simulink model "variacion_tau"  (R2026a)
settings: Solver=VariableStepAuto
values from neighbouring files (symbols this model uses):
  K = cambio_y / delta_u    [Taller_1_Identificacion_grafica_de_sistemas_FOTD.m]
  t_escalon = t(idx_escalon + 1)    [Taller_1_Identificacion_grafica_de_sistemas_FOTD.m]
  tau_analitico = 1.5 * (t_63_relativo - t_28_relativo)    [Taller_1_Identificacion_grafica_de_sistemas_FOTD.m]
  theta_analitico = t_63_relativo - tau_analitico    [Taller_1_Identificacion_grafica_de_sistemas_FOTD.m]
settings Model: Creator=Daniel  LastModifiedBy=Daniel

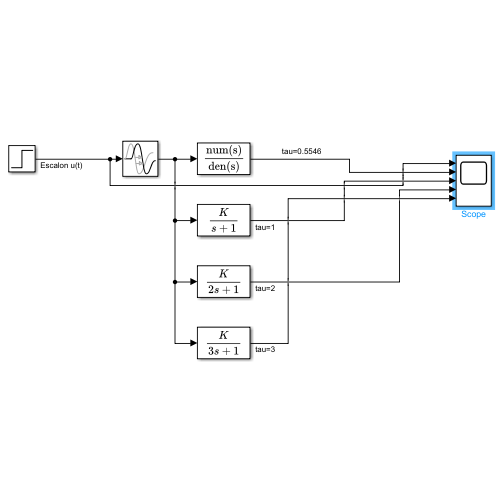
[thumbnail: Simulink's stored preview of the top-level diagram]
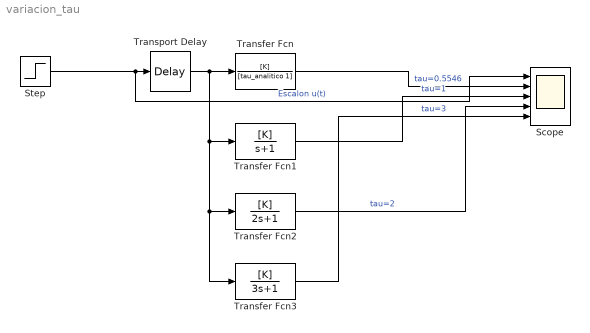
== system variacion_tau ==
  Scope : Scope  NumInputPorts=5
      settings: Title=Respuesta del Modelo Analítico  ActiveDisplayYMinimum=-0.4882625489147906  ActiveDisplayYMaximum=2.634836077109187  YLabel=Amplitud
  Step : Step  Time=t_escalon  FinalValue=1.5  SampleTime=0
  Transfer Fcn : TransferFcn  Numerator=[K]  Denominator=[tau_analitico 1]
  Transfer Fcn1 : TransferFcn  Numerator=[K]  Denominator=[1 1]
  Transfer Fcn2 : TransferFcn  Numerator=[K]  Denominator=[2 1]
  Transfer Fcn3 : TransferFcn  Numerator=[K]  Denominator=[3 1]
  Transport Delay : TransportDelay  DelayTime=theta_analitico
  wires:
  Transfer Fcn2/1 -> Scope/4  "tau=2"
  Transfer Fcn1/1 -> Scope/3  "tau=1"
  Transfer Fcn3/1 -> Scope/5  "tau=3"
  Step/1 -> Scope/1, Transport Delay/1  "Escalon u(t)"
  Transfer Fcn/1 -> Scope/2  "tau=0.5546"
  Transport Delay/1 -> Transfer Fcn3/1, Transfer Fcn2/1, Transfer Fcn1/1, Transfer Fcn/1
